simulink model "Q5"  (R2016a)
settings: Solver=VariableStepAuto  StartTime=0.0  StopTime=10.0  RelTol=1e-3
settings Model: Creator=duyvu  LastModifiedBy=duyvu

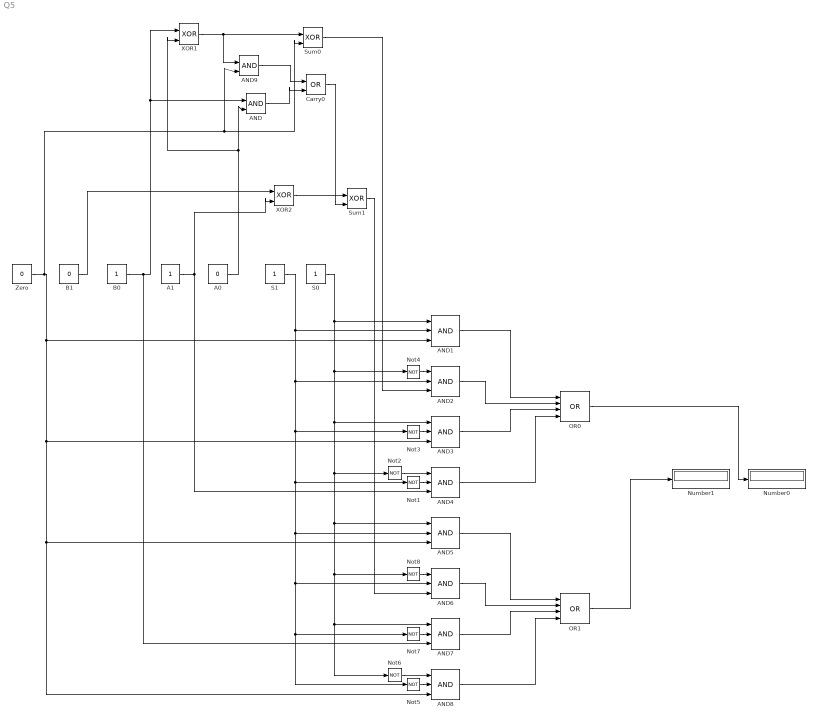
== system Q5 ==
  A0 : Constant  Value=0  OutDataTypeStr=boolean
  A1 : Constant  OutDataTypeStr=boolean
  AND : Logic  IconShape=distinctive  AllPortsSameDT=off  OutDataTypeStr=boolean
  AND{1..8} (8 alike) : Logic  Inputs=3  IconShape=distinctive  AllPortsSameDT=off  OutDataTypeStr=boolean
  AND9 : Logic  IconShape=distinctive  AllPortsSameDT=off  OutDataTypeStr=boolean
  B0 : Constant  OutDataTypeStr=boolean
  B1 : Constant  Value=0  OutDataTypeStr=boolean
  "Carry0 " : Logic  Operator=OR  IconShape=distinctive  AllPortsSameDT=off  OutDataTypeStr=boolean
  Not{1..8} (8 alike) : Logic  Operator=NOT  Inputs=3  IconShape=distinctive  AllPortsSameDT=off  OutDataTypeStr=boolean
  Number0 : Display
  Number1 : Display
  OR0 : Logic  Operator=OR  Inputs=4  IconShape=distinctive  AllPortsSameDT=off  OutDataTypeStr=boolean
  OR1 : Logic  Operator=OR  Inputs=4  IconShape=distinctive  AllPortsSameDT=off  OutDataTypeStr=boolean
  S0 : Constant  OutDataTypeStr=boolean
  S1 : Constant  OutDataTypeStr=boolean
  Sum0 : Logic  Operator=XOR  IconShape=distinctive  AllPortsSameDT=off  OutDataTypeStr=boolean
  Sum1 : Logic  Operator=XOR  IconShape=distinctive  AllPortsSameDT=off  OutDataTypeStr=boolean
  XOR1 : Logic  Operator=XOR  IconShape=distinctive  AllPortsSameDT=off  OutDataTypeStr=boolean
  XOR2 : Logic  Operator=XOR  IconShape=distinctive  AllPortsSameDT=off  OutDataTypeStr=boolean
  Zero : Constant  Value=0  OutDataTypeStr=boolean
  wires:
  AND1/1 -> OR0/1
  AND2/1 -> OR0/2
  AND3/1 -> OR0/3
  AND4/1 -> OR0/4
  AND5/1 -> OR1/1
  AND6/1 -> OR1/2
  AND7/1 -> OR1/3
  AND8/1 -> OR1/4
  S0/1 -> Not6/1, AND7/1, Not8/1, AND5/1, Not2/1, AND3/1, Not4/1, AND1/1
  S1/1 -> AND1/2, AND2/2, Not3/1, Not1/1, AND5/2, AND6/2, Not7/1, Not5/1
  Not1/1 -> AND4/2
  Not2/1 -> AND4/1
  Not3/1 -> AND3/2
  Not4/1 -> AND2/1
  Not5/1 -> AND8/2
  Not6/1 -> AND8/1
  Not7/1 -> AND7/2
  Not8/1 -> AND6/1
  Zero/1 -> Sum0/2, AND9/2, AND1/3, AND5/3, AND8/3, AND3/3
  XOR1/1 -> AND9/1, Sum0/1
  AND9/1 -> "Carry0 "/1
  AND/1 -> "Carry0 "/2
  OR0/1 -> Number0/1
  OR1/1 -> Number1/1
  A1/1 -> XOR2/2, AND4/3
  B0/1 -> AND7/3, AND/1, XOR1/1
  A0/1 -> XOR1/2, AND/2
  Sum0/1 -> AND2/3
  XOR2/1 -> Sum1/1
  "Carry0 "/1 -> Sum1/2
  B1/1 -> XOR2/1
  Sum1/1 -> AND6/3
